simulink model "chap5_6sim"  (Simulink 5.0)
settings: Solver=ode45  StartTime=0.0  StopTime=1  FixedStep=0.001  RelTol=1e-5  AbsTol=1e-5
PreLoadFcn:
  | i=k;
settings Model: LastModifiedBy=Administrator  MaxDataPoints=10000  RTWOptions="-aEnforceIntegerDowncast=1 -aExtMode=0 -aExtModeTesting=0 -aFoldNonRolledExpr=1 -aForceParamTrailComments=0 -aGenerateComments=1 -aGenerateReport=0 -aIgnoreCustomStorageClasses=1 -aIncDataTypeInIds=0 -aIncHierarchyInIds=0 -aInlineInvariantSignals=0 -aInlinedPrmAccess=\"Literals\" -aLocalBlockOutputs=1 -aLogVarNameModifier=\"rt_\" -aMaxRTWIdLen=31 -aPrefixModelToSubsysFcnNames=1 -aRTWVerbose=1 -aRollThreshold=5 -aShowEliminatedStatements=0"

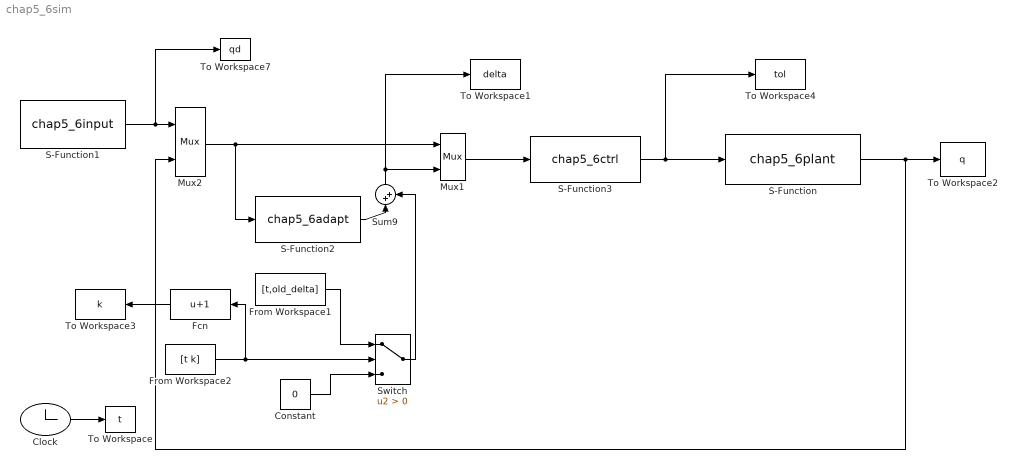
== system chap5_6sim ==
  Clock : Clock
      settings: Decimation=10
  Constant : Constant  Value=0
  Fcn : Fcn  Orientation=left  Expr=u+1
  From Workspace1 : FromWorkspace  VariableName=[t,old_delta]  SampleTime=0
  From Workspace2 : FromWorkspace  VariableName=[t k]  SampleTime=0
  Mux1 : Mux  Inputs=2
  Mux2 : Mux  Inputs=2
  S-Function : S-Function  FunctionName=chap5_6plant
  S-Function1 : S-Function  FunctionName=chap5_6input
  S-Function2 : S-Function  FunctionName=chap5_6adapt
  S-Function3 : S-Function  FunctionName=chap5_6ctrl
  Sum9 : Sum  Orientation=up  Inputs=|++  SaturateOnIntegerOverflow=on
  Switch : Switch  Criteria=u2 > Threshold  SaturateOnIntegerOverflow=on
  To Workspace : ToWorkspace  VariableName=t  SampleTime=-1  SaveFormat=Array
  To Workspace1 : ToWorkspace  VariableName=delta  SampleTime=-1  SaveFormat=Array
  To Workspace2 : ToWorkspace  VariableName=q  SampleTime=-1  SaveFormat=Array
  To Workspace3 : ToWorkspace  VariableName=k  SampleTime=-1  SaveFormat=Array
  To Workspace4 : ToWorkspace  VariableName=tol  SampleTime=-1  SaveFormat=Array
  To Workspace7 : ToWorkspace  VariableName=qd  SampleTime=-1  SaveFormat=Array
  wires:
  S-Function/1 -> To Workspace2/1, Mux2/2
  Clock/1 -> To Workspace/1
  S-Function1/1 -> To Workspace7/1, Mux2/1
  S-Function2/1 -> Sum9/1
  Sum9/1 -> To Workspace1/1, Mux1/2
  Switch/1 -> Sum9/2
  Constant/1 -> Switch/3
  Mux2/1 -> S-Function2/1, Mux1/1
  From Workspace1/1 -> Switch/1
  From Workspace2/1 -> Switch/2, Fcn/1
  S-Function3/1 -> S-Function/1, To Workspace4/1
  Mux1/1 -> S-Function3/1
  Fcn/1 -> To Workspace3/1
